simulink model "TxRx"  (R2021a)
settings: Solver=FixedStepDiscrete  StartTime=0.0  StopTime=10000  RelTol=1e-3
libraries: commrandsrc3 x1
settings Model: Creator=Mustafa  LastModifiedBy=Mustafa
settings OptimizationCC: DefaultParameterBehavior=Inlined  UseDivisionForNetSlopeComputation=on  GainParamInheritBuiltInType=on  UseFloatMulNetSlope=on  InlineInvariantSignals=on  PassReuseOutputArgsAs=Individual arguments  ZeroExternalMemoryAtStartup=off  ZeroInternalMemoryAtStartup=off  NoFixptDivByZeroProtection=on  EfficientFloat2IntCast=on  LifeSpan=1  OptimizeBlockOrder=speed  DifferentSizesBufferReuse=on  EfficientTunableParamExpr=on
settings DebuggingCC: ParameterTunabilityLossMsg=error
settings HardwareCC: ProdLongLongMode=on
settings SFSimCC: MATLABDynamicMemAlloc=off
settings RTWCC: SystemTargetFile=ert.tlc  TemplateMakefile=ert_default_tmf
settings CodeAppCC: ForceParamTrailComments=on  IgnoreCustomStorageClasses=off  OperatorAnnotations=on  SimulinkDataObjDesc=on  SFDataObjDesc=on  CustomSymbolStrGlobalVar=rt$N$M  CustomSymbolStrType=$N$M  CustomSymbolStrFcn=$N$M$F  CustomSymbolStrMacro=$N$M  InsertBlockDesc=on
settings ERTTargetCC: TargetLangStandard=C99 (ISO)  GenerateSampleERTMain=on  IncludeMdlTerminateFcn=off  CombineSignalStateStructs=on  SuppressErrorStatus=on  SupportAbsoluteTime=off  SupportComplex=off  InlinedParameterPlacement=NonHierarchical  ERTCustomFileTemplate=example_file_process.tlc  ERTFilePackagingFormat=CompactWithDataFile

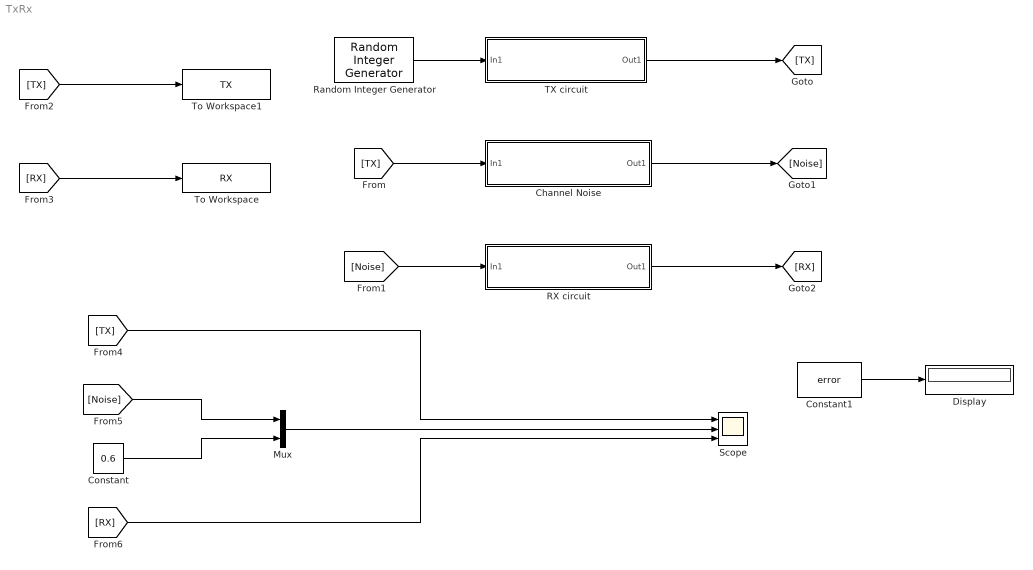
== system TxRx ==
  Channel Noise : Subsystem
  Constant : Constant  Value=0.6
  Constant1 : Constant  Value=error
  Display : Display
  Mux : Mux  Inputs=2
  RX circuit : Subsystem
  Random Integer Generator : commrandsrc3/Random Integer Generator  SetSize=2  SeedSource=Auto  Seed=0  SampleTime=1  SamplesPerFrame=1  OutputDataType=boolean  SimulateUsing=Interpreted execution
  Scope : Scope  NumInputPorts=3
  TX circuit : Subsystem
  To Workspace : ToWorkspace  VariableName=RX  SampleTime=-1
      settings: Save2DSignal=2-D array (concatenate along first dimension)
  To Workspace1 : ToWorkspace  VariableName=TX  SampleTime=-1
      settings: Save2DSignal=2-D array (concatenate along first dimension)
  wires:
  Random Integer Generator/1 -> TX circuit/1(In1)
  TX circuit/1(Out1) -> [TX]
  [TX] -> Channel Noise/1(In1)
  Channel Noise/1(Out1) -> [Noise]
  [Noise] -> RX circuit/1(In1)
  RX circuit/1(Out1) -> [RX]
  [TX] -> To Workspace1/1
  [RX] -> To Workspace/1
  [TX] -> Scope/1
  [RX] -> Scope/3
  [Noise] -> Mux/1
  Constant/1 -> Mux/2
  Mux/1 -> Scope/2
  Constant1/1 -> Display/1

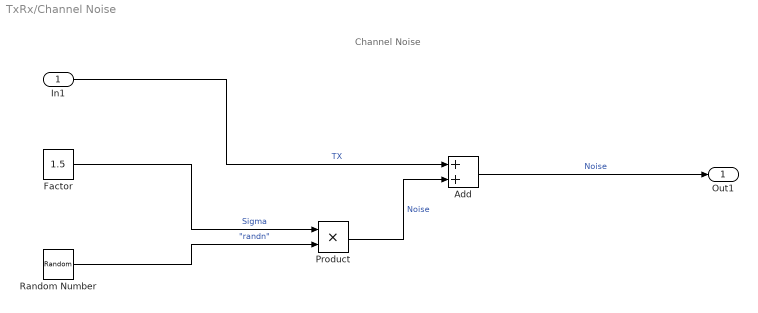
== system TxRx/Channel Noise ==
  note: Channel Noise
  In1 : Inport
  Add : Sum
  Factor : Constant  Value=1.5
  Product : Product
  Random Number : RandomNumber  SampleTime=1
  Out1 : Outport
  wires:
  In1/1 -> Add/1  "TX"
  Product/1 -> Add/2  "Noise"
  Factor/1 -> Product/1  "Sigma"
  Random Number/1 -> Product/2  "\"randn\""
  Add/1 -> Out1/1  "Noise"

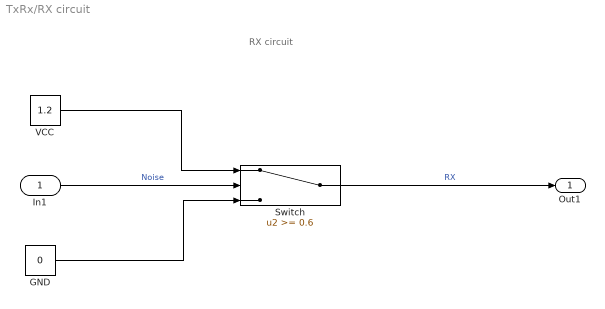
== system TxRx/RX circuit ==
  note: RX circuit
  In1 : Inport
  GND : Constant  Value=0
  Switch : Switch  Threshold=0.6
  VCC : Constant  Value=1.2
  Out1 : Outport
  wires:
  In1/1 -> Switch/2  "Noise"
  VCC/1 -> Switch/1
  GND/1 -> Switch/3
  Switch/1 -> Out1/1  "RX"

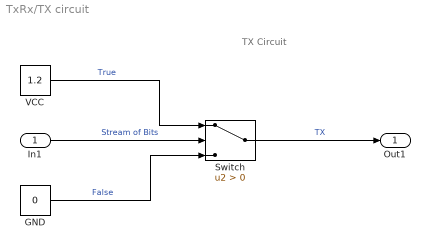
== system TxRx/TX circuit ==
  note: TX Circuit
  In1 : Inport
  GND : Constant  Value=0
  Switch : Switch  Criteria=u2 > Threshold
  VCC : Constant  Value=1.2
  Out1 : Outport
  wires:
  In1/1 -> Switch/2  "Stream of Bits"
  GND/1 -> Switch/3  "False"
  VCC/1 -> Switch/1  "True"
  Switch/1 -> Out1/1  "TX"
